simulink model "QpskTxBradeRf"  (R2015b)
settings: Solver=VariableStepAuto  StartTime=0.0  StopTime=inf  RelTol=1e-3
libraries: dspsigops x1, commsequence2 x1, commdigbbndpm3 x1, commfilt2 x1
settings Model: ModifiedByFormat=RapidRadio  Creator=RapidRadio  LastModifiedBy=RapidRadio

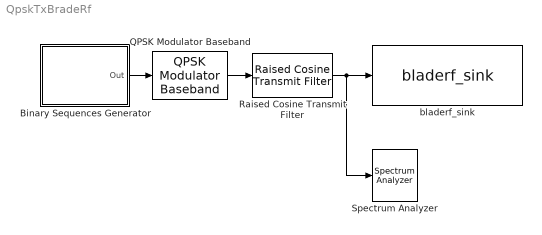
== system QpskTxBradeRf ==
  Binary Sequences Generator : Subsystem
      mask Display: disp('Binary Sequences\nGenerator')
  QPSK Modulator Baseband : commdigbbndpm3/QPSK Modulator Baseband  InType=Bit  Enc=Gray  Ph=pi/4  outDtype=double  outWordLen=16  outUDDataType=sfix(16)  outFracLenMode=Best precision  outFracLen=15
  Raised Cosine Transmit Filter : commfilt2/Raised Cosine Transmit Filter  filtType=Square root  filtSpan=10  currentFiltSpan=10  D=(10)/2  R=0.5  sampMode=Mute  saveAsFlag=0  N=8  framing=Enforce single-rate processing  InputProcessing=Columns as channels (frame based)  checkGain=Normalized  filterGain=1  checkCoeff=off  variableName=rcTxFilt1  launchFVT=off  roundingMode=Floor  overflowMode=off
  Spectrum Analyzer : SpectrumAnalyzer
  bladerf_sink : S-Function  FunctionName=bladerf_sink  Parameters=set_index,samplerate,set_bandwidth,set_freq,set_txvga1,set_txvga2,set_frame,set_frame_type  SFunctionDeploymentMode=off  EnableBusSupport=off  mask(bladeRF Sink){bladerf_device_index=0, bladerf_query=on, bladerf_samplerate=2e6, bladerf_lpf=1.75 MHz, bladerf_frame_length=888, bladerf_frame_type=Frame, bladerf_frequency=2.4e9, bladerf_txvga1=-4, bladerf_txvga2=5, bladerf_restore_block=off}
      mask prompts: bladerf_device_index "Device Index:"; bladerf_query "Find Devices (click, see MATLAB console output)"; bladerf_samplerate "Sample Rate (SPS):"; bladerf_lpf "Low Pass Filter Bandwith"; bladerf_frame_length "Samples per frame"; bladerf_frame_type "Output Type"; bladerf_frequency "Carrier Frequency (Hz):"; bladerf_txvga1 "TXVGA1 Gain (dB)"; bladerf_txvga2 "TXVGA2 Gain (dB)"; bladerf_restore_block "Restore Block Size (click)"
      mask help: Transmit data to a bladeRF device.
      mask init:
      | % initialize
      | % S-params set_index,samplerate,set_bandwidth,set_freq,set_lnagain,set_rxvga1,set_rxvga2,set_frame,set_frame_type
      | mask_display_text = [];
      | 
      | port=0;
      | 
      | % check identifier
      | if (isreal(bladerf_device_index) && bladerf_device_index >= 0)
      |     set_index=bladerf_device_index;
      | else
      |     error('The device index must be a number greater or equal 0 !!!')
      | end
      | 
      | % mask display device index
      | if strcmp(get_param(gcb,'bladerf_device_index'),' ')
      |     mask_display_text = [mask_display_text 'disp(''No Device'');'];
      | else
      |     mask_display_text = [mask_display_text 'disp(''bladeRF #' num2str(bladerf_device_index) ''');'];
      | end
      | if (bladerf_samplerate < bladerf_lpf)
      |     warning('The bandwidth should be lower than the samplerate, use with caution')
      | end
      | % check samplerate
      | if (isreal(bladerf_samplerate))
      |     if (bladerf_samplerate > 0)
      |         samplerate=uint32(bladerf_samplerate);
      |         if (samplerate ~= bladerf_samplerate)
      |             fprintf('Sample Rate adjusted to %u Sps\n',samplerate);
      |         end
      |     else
      |         error('The samplerate has to be greater than 0 !!!')
      |     end
      | else
      |     error('The samplerate has to be number !!!')
      | end
      | 
      | bws = [28e6 20e6 14e6 12e6 8.75e6 7e6 6e6 5.5e6 5e6 3.84e6 3e6 2.75e6 2.5e6 1.75e6 1.5e6];
      | set_bandwidth = bws(bladerf_lpf);
      | if (set_bandwidth > bladerf_samplerate)
      |     warning('Sampling rate (Sps) should be equal to or greater than Low Pass Filter Bandwidth to satisfy Nyquist sampling rate');
      | end
      | 
      | % check frequency
      | if (isreal(bladerf_frequency) && bladerf_frequency >= 0)
      |         set_freq=uint32(bladerf_frequency);
      |         if (set_freq ~= bladerf_frequency)
      |                 fprintf('Frequency adjusted to %d\n',set_freq);
      |         end
      | else
      |     error('The frequency has to be number greater than 0 !!!')
      | end
      | 
      | % RXVGA1
      | if (isreal(bladerf_txvga1))
      |     if (bladerf_txvga1 < -35)
      |         error('TXVGA1 Gain has to be greater than or equal to -35dB\n');
      |     elseif (bladerf_txvga1 > -4)
      |         error('TXVGA1 Gain has to be less than or equal to -4dB\n');
      |     else
      |         set_txvga1 = uint32(bladerf_txvga1);
      |         if (set_txvga1 ~= bladerf_txvga1)
      |             fprintf('TXVGA1 Gain set to %u dB\n', set_txvga1)
      |         end
      |     end
      | end
      | 
      | % RXVGA2
      | if (isreal(bladerf_txvga2))
      |     if (bladerf_txvga2 < 0)
      |         error('TXVGA2 Gain has to be greater than or equal to 0dB\n');
      |     elseif (bladerf_txvga2 > 25)
      |         error('TXVGA2 Gain has to be less than or equal to 25dB\n');
      |     else
      |         set_txvga2 = uint32(bladerf_txvga2);
      |         if (set_txvga2 ~= bladerf_txvga2)
      |             fprintf('TXVGA2 Gain set to %u dB\n', set_txvga2)
      |         end
      |     end
      | end
      | 
      | % check frame length
      | if (isreal(bladerf_frame_length) && bladerf_frame_length > 0)
      |     set_frame=bladerf_frame_length;
      | else
      |     error('The frame length has to be number greater than 0 !!!')
      | end
      | 
      | % check frame type
      | if (strcmp(get_param(gcb,'bladerf_frame_type'),'Frame'))
      |     % use frames
      |     set_frame_type=1;
      | else
      |     % use vectors
      |     set_frame_type=0;
      | end
      |     
      | % set mask display
      | set_param(gcb,'MaskDisplay',mask_display_text);
      mask Help: web(fullfile(bladerf_get_path, 'blockset', 'bladerf_sink.html'), '-helpbrowser')
      mask TypeOptions bladerf_lpf: 28 MHz | 20 MHz | 14 Mhz | 12 Mhz | 8.75 Mhz | 7 MHz | 6 Mhz | 5.5 MHz | 5 MHz | 3.84 MHz | 3 MHz | 2.75 MHz | 2.5 MHz | 1.75 MHz | 1.5 MHz
      mask TypeOptions bladerf_frame_type: Frame | Vector
      mask Callback bladerf_restore_block:
      | % restore block size
      | block_width=150;
      | block_height=60;
      | 
      | if strcmp(get_param(gcb,'bladerf_restore_block'),'on')
      |    pos=get_param(gcb,'Position');
      |    pos=[pos(1) pos(2) pos(1)+block_width pos(2)+block_height];
      |    set_param(gcb,'Position',pos);
      | end
      | 
      | set_param(gcb,'bladerf_restore_block','off');
      | 
      | clear pos block_width block_height
      mask Display: disp('bladeRF #0');
  wires:
  Binary Sequences Generator/1(Out) -> QPSK Modulator Baseband/1
  QPSK Modulator Baseband/1 -> Raised Cosine Transmit Filter/1
  Raised Cosine Transmit Filter/1 -> Spectrum Analyzer/1, bladerf_sink/1

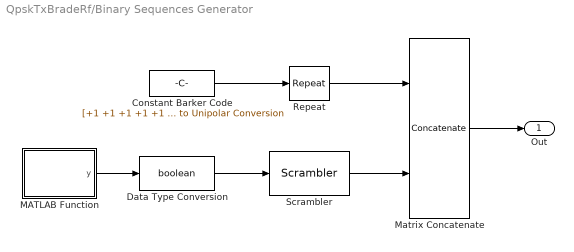
== system QpskTxBradeRf/Binary Sequences Generator ==
  Constant Barker Code : Constant  Value=|  VectorParams1D=off  OutDataTypeStr=boolean  SampleTime=1  FramePeriod=888/2e6
      | [+1 +1 +1 +1 +1 -1 -1 +1 +1 -1 +1 -1 +1
      | ].' > 0  % Bipolar to Unipolar Conversion
      settings: SamplingMode=Frame based
  Data Type Conversion : DataTypeConversion  OutDataTypeStr=boolean
  MATLAB Function : MATLAB Function  TreatAsAtomicUnit=on
  Matrix Concatenate : Concatenate  Mode=Multidimensional array
  Repeat : dspsigops/Repeat  N=2  InputProcessing=Columns as channels (frame based)  RateOptions=Enforce single-rate processing  ic=0  mode=Unused parameter value
  Scrambler : commsequence2/Scrambler  M=2  poly=[1 1 1 0 1]  iniStaSource=Dialog Parameter  ini_sta=[0 0 0 0]  resetViaPort=off
  Out : Outport
  wires:
  Matrix Concatenate/1 -> Out/1
  Repeat/1 -> Matrix Concatenate/1
  Data Type Conversion/1 -> Scrambler/1
  MATLAB Function/1(y) -> Data Type Conversion/1
  Constant Barker Code/1 -> Repeat/1
  Scrambler/1 -> Matrix Concatenate/2

== matlab function QpskTxBradeRf/Binary Sequences Generator/MATLAB Function ==
  data: y output
function y = fcn()
% Generate a sequence of binary numbers

% String of a payload
string = 'This is a QPSK Transmitter';

% Convert to a sequence of binary numbers
binary = de2bi(int8(string),7,'left-msb');
y_buf = reshape(binary, [numel(binary) 1]);

% Add 2bits in order to divide a payload including a sequence of Barcar
% codes by 2(QPSK: 2bits/symbol) without a remainder.
y = [y_buf ; 0 ; 0 ; 0 ; 0 ; 0 ; 0 ; 0 ; 0 ; 0 ; 0 ; 0 ; 0 ; 0 ; 0];
